simulink model "sscv_braking_ABS_w_vehicle"  (R2024a)
settings: Solver=ode23t  StartTime=0.0  StopTime=1  RelTol=1e-3  AbsTol=1e-3
PreLoadFcn:
  | sscv_braking_ABS_w_vehicle_input
values from neighbouring files (symbols this model uses):
  wheel_rad = 0.3    [sscv_braking_ABS_w_vehicle_input.m]
  wheel_vth = 0.01    [sscv_braking_ABS_w_vehicle_input.m]
undefined symbols (not defined in the file or in its folder): Asphalt, fcdb, HCU, MFormulaCoeff, tpc, vb
libraries: fl_lib x165, SimscapeFluids_lib x24, nesl_utility x21, sdl_lib x9, simulink x3, simulink_extras x1
(part 1 of 6)
CloseFcn:
  | clear brkTs fcdb HCU MFormulaCoeff mu period
  | clear simlog_sscv_braking_ABS_w_vehicle
  | clear Slip tpc tout vb wheel_rad wheel_vth
  | 
  | try,close(h_sscv_braking_ABS_w_vehicle),end
  | clear h_sscv_braking_ABS_w_vehicle
Description:
  | Anti-Lock Braking System (ABS)
settings Model: Creator=The MathWorks, Inc.  LastModifiedBy=The MathWorks, Inc.
settings SolverCC: AutoScaleAbsTol=off  MaxConsecutiveMinStep=10  ZeroCrossAlgorithm=Adaptive  AlgebraicLoopSolver=TrustRegion
settings DataIOCC: SignalLogging=off  ReturnWorkspaceOutputs=off
settings OptimizationCC: ReuseModelBlockBuffer=off
settings DebuggingCC: MaskedZcDiagnostic=none  IgnoredZcDiagnostic=none  UnconnectedInputMsg=warning  UnconnectedOutputMsg=warning  UnconnectedLineMsg=warning
settings ModelReferenceCC: EnableRefExpFcnMdlSchedulingChecks=on
settings RTWCC: GPUComputeCapability=3.5  DLArmComputeVersion=19.05
settings SimscapeCC: SimscapeLogType=all  SimscapeLogName=simlog_sscv_braking_ABS_w_vehicle  SimscapeLogLimitData=off

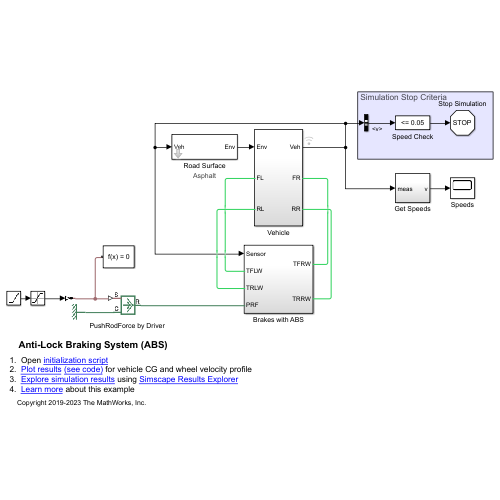
[thumbnail: Simulink's stored preview of the top-level diagram]
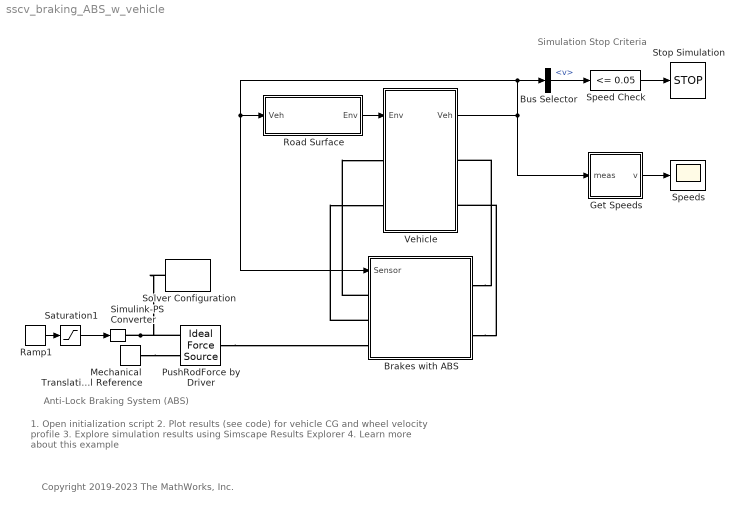
== system sscv_braking_ABS_w_vehicle ==
  note: Anti-Lock Braking System (ABS)
  note: 1. Open initialization script
      | 2. Plot results (see code) for vehicle CG and wheel velocity profile
      | 3. Explore simulation results using Simscape Results Explorer
      | 4. Learn more about this example
  note: Simulation Stop Criteria
  note: Copyright 2019-2023 The MathWorks, Inc.
  Brakes with ABS : Subsystem
  Bus Selector : BusSelector  OutputSignals=v
  Get Speeds : Subsystem
  Mechanical Translational Reference : fl_lib/Mechanical/Translational Elements/Mechanical Translational Reference
  PushRodForce by Driver : fl_lib/Mechanical/Mechanical Sources/Ideal Force Source
  Ramp1 : simulink/Sources/Ramp  slope=tpc.pushRodF(3)*10  start=0.1  InitialOutput=0
  Road Surface : Subsystem  mask{road_condition=Asphalt}
      mask prompts: road_condition "Road Condition"
      settings: AttributesFormatString=%<road_condition>
      mask TypeOptions road_condition: Road/road_condition
  Saturation1 : Saturate  UpperLimit=tpc.pushRodF(3)  LowerLimit=0
  Simulink-PS Converter : nesl_utility/Simulink-PS Converter  PhysicalDomain=network_engine_domain  SubClassName=ps_input  LeftPortType=input  RightPortType=output  PseudoPeriodic=off  Frequencies=[]  NoiseDistribution=none  NoiseParameters=[]  Unit=1  AffineConversion=off  FilteringAndDerivatives=filter  SimscapeFilterOrder=1  InputFilterTimeConstant=0.001  UdotUserProvided=0
  Solver Configuration : nesl_utility/Solver Configuration  Tag=ModelFeatures  PhysicalDomain=network_engine_domain  SubClassName=solver  LeftPortType=input  RightPortType=generic  Tones=[]  Harmonics=[]  SimulateNoise=off  Profile=off  UseLocalSampling=off  EnableSwitchedLinearOptims=on  FrequencyDomain=off  UseCCode=off  RelTol=0.001  AbsTol=1e-06  MinStep=1e-09  ToWorkspace=off  RevertToSquareIcSolve=off  NumHomotopyIterations=100  PhasorMode=off  PhasorModeNumHarmonics=1  ConsistencySolver=NEWTON_FTOL  IndexReductionMethod=DerivativeReplacement  DoDC=off  ResidualTolerance=1e-09  ConsistencyTolSource=GLOBAL  ConsistencyAbsTol=0.001  ConsistencyRelTol=0.001  ConsistencyTolFactor=0.001  UseLocalSolver=off  LocalSolverChoice=NE_BACKWARD_EULER_ADVANCER  ResolveIndetEquations=on  FunctionEvalNumThread=1  LocalSolverSampleTime=0.001  DoFixedCost=off  MaxNonlinIter=3  MaxModeIter=2  ComputeImpulses=off  ImpulseIterations=1  LinearAlgebra=auto  LinearAlgebraNumThread=0  EquationFormulation=NE_TIME_EF  DelaysMemoryBudget=1024  AutomaticFiltering=on  FilteringTimeConstant=0.001  PartitionStorageMethod=AS_NEEDED  PartitionMemoryBudget=1024  PartitionMethod=FAST  MultibodyUseLocalSolver=off  MultibodyLocalSolverChoice=ODE1  MultibodyLocalSolverSampleTime=0.001
  Speed Check : simulink/Logic and Bit Operations/Compare To Constant  relop=<=  const=0.05  OutDataTypeStr=boolean
  Speeds : Scope
  Stop Simulation : Stop
  Vehicle : Subsystem
  wires:
  Speed Check/1 -> Stop Simulation/1
  Vehicle/1(Veh) -> Brakes with ABS/1(Sensor), Road Surface/1(Veh), Bus Selector/1, Get Speeds/1(meas)
  Road Surface/1(Env) -> Vehicle/1(Env)
  Bus Selector/1 -> Speed Check/1  "<v>"
  Get Speeds/1(v) -> Speeds/1
  Ramp1/1 -> Saturation1/1
  Saturation1/1 -> Simulink-PS Converter/1
  connections:
  Brakes with ABS/LConn1 -- Vehicle/LConn1
  Brakes with ABS/RConn1 -- Vehicle/RConn1
  Brakes with ABS/LConn2 -- Vehicle/LConn2
  Brakes with ABS/RConn2 -- Vehicle/RConn2
  Simulink-PS Converter/RConn1 -- PushRodForce by Driver/RConn1 -- Solver Configuration/RConn1
  PushRodForce by Driver/LConn1 -- Brakes with ABS/LConn3
  Mechanical Translational Reference/LConn1 -- PushRodForce by Driver/RConn2

== system sscv_braking_ABS_w_vehicle/Brakes with ABS ==
  note: Fixed Caliper Disc Brakes
  Sensor : Inport
  ABS : Subsystem
  FCDB : Subsystem  Tag=ModelFeatures
  Vacuum Boosted Tandem Primary Cylinder : Subsystem
  TFLW : PMIOPort  Side=Left
  TFRW : PMIOPort  Port=2  Side=Right
  TRLW : PMIOPort  Port=3  Side=Left
  TRRW : PMIOPort  Port=4  Side=Right
  PRF : PMIOPort  Port=5  Side=Left
  wires:
  Sensor/1 -> ABS/1(Sensor)
  connections:
  ABS/LConn3 -- Vacuum Boosted Tandem Primary Cylinder/LConn1
  FCDB/LConn3 -- ABS/LConn1
  FCDB/RConn2 -- TRRW/RConn1
  ABS/LConn2 -- FCDB/LConn4
  ABS/RConn2 -- FCDB/RConn4
  FCDB/RConn3 -- ABS/RConn1
  ABS/RConn3 -- Vacuum Boosted Tandem Primary Cylinder/RConn1
  FCDB/RConn1 -- TFRW/RConn1
  FCDB/LConn1 -- TFLW/RConn1
  FCDB/LConn2 -- TRLW/RConn1
  PRF/RConn1 -- Vacuum Boosted Tandem Primary Cylinder/LConn2

== system sscv_braking_ABS_w_vehicle/Get Speeds ==
  meas : Inport
  Bus Selector2 : BusSelector  OutputSignals=v,FL.v,FR.v,RL.v,RR.v
  Demux : Demux  Outputs=5
  Mux : Mux  Inputs=5
  Mux1 : Mux  Inputs=5
  v : Outport  VectorParamsAs1DForOutWhenUnconnected=off
  wires:
  Bus Selector2/4 -> Mux/4  "<v>"
  Bus Selector2/3 -> Mux/3  "<v>"
  Bus Selector2/2 -> Mux/2  "<v>"
  Bus Selector2/5 -> Mux/5  "<v>"
  meas/1 -> Bus Selector2/1
  Bus Selector2/1 -> Mux/1  "<v>"
  Mux/1 -> Demux/1
  Mux1/1 -> v/1
  Demux/1 -> Mux1/1  "Vehicle CG  velocity"
  Demux/2 -> Mux1/2  "Front left tire velocity"
  Demux/3 -> Mux1/3  "Front right tire velocity"
  Demux/4 -> Mux1/4  "Rear left tire velocity"
  Demux/5 -> Mux1/5  "Rear right tire velocity"

== system sscv_braking_ABS_w_vehicle/Road Surface ==
  In Bus Element : Inport  PortName=Veh  Element=x
  Bus Creator : BusCreator  Inputs=3
  Bus Creator1 : BusCreator  Inputs=4
  Constant : Constant  Value=0
  Constant1 : Constant  Value=0
  Road : Subsystem  mask(Testing Surface){road_condition=Asphalt, surface_LF=0, surface_RF=0, surface_LR=0, surface_RR=0, surface_xpos=0}
      mask prompts: road_condition "Road Condition"; surface_LF "Surface LF"; surface_RF "Surface RF"; surface_LR "Surface LR"; surface_RR "Surface RR"; surface_xpos "Surface Position"
      mask help: Select surface for test. Specifies locations of high and low friction surface as a function of longitudinal distance for each tire.
      mask init:
      | if (road_condition==1)
      |     % Road: low coeff to high coeff
      |     surface_LF   = [3 1 1 3 3];
      |     surface_RF   = [3 1 1 3 3];
      |     surface_LR   = [3 1 1 3 3];
      |     surface_RR   = [3 1 1 3 3];
      |     surface_xpos = [-1 0 24.9 25 26]+6;
      | elseif(road_condition==2)
      |     % Road: Split (low left side)
      |     surface_LF   = [1 1 1 1 1];
      |     surface_RF   = [4 4 4 4 4];
      |     surface_LR   = [1 1 1 1 1];
      |     surface_RR   = [4 4 4 4 4];
      |     surface_xpos = [-1 0 4.9 5 6];
      | elseif(road_condition==3)
      |     % Road: Asphalt
      |     surface_LF   = [4 4 4 4 4];
      |     surface_RF   = [4 4 4 4 4];
      |     surface_LR   = [4 4 4 4 4];
      |     surface_RR   = [4 4 4 4 4];
      |     surface_xpos = [-1 0 4.9 5 6];
      | elseif(road_condition==4)
      |     % Road: Wet Asphalt
      |     surface_LF   = [3 3 3 3 3];
      |     surface_RF   = [3 3 3 3 3];
      |     surface_LR   = [3 3 3 3 3];
      |     surface_RR   = [3 3 3 3 3];
      |     surface_xpos = [-1 0 4.9 5 6];
      | elseif(road_condition==5)
      |     % Road: Ice
      |     surface_LF   = [1 1 1 1 1];
      |     surface_RF   = [1 1 1 1 1];
      |     surface_LR   = [1 1 1 1 1];
      |     surface_RR   = [1 1 1 1 1];
      |     surface_xpos = [-1 0 4.9 5 6];
      | end
      settings: AttributesFormatString=%<road_condition>
      mask TypeOptions road_condition: Transition: Low to high mu | Split: Low mu on left | Asphalt | Wet Asphalt | Ice
  Env : Outport  VectorParamsAs1DForOutWhenUnconnected=off
  wires:
  Constant1/1 -> Bus Creator/2  "Slope"
  Constant/1 -> Bus Creator/1  "Wind"
  Bus Creator/1 -> Env/1  "Env"
  Road/1(FL) -> Bus Creator1/1  "FL"
  Road/2(FR) -> Bus Creator1/2  "FR"
  Road/3(RL) -> Bus Creator1/3  "RL"
  Road/4(RR) -> Bus Creator1/4  "RR"
  Bus Creator1/1 -> Bus Creator/3  "mu"
  In Bus Element/1 -> Road/1(wX)

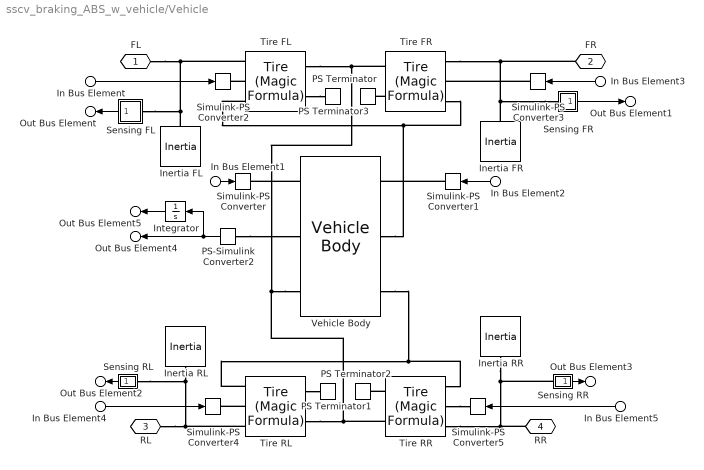
== system sscv_braking_ABS_w_vehicle/Vehicle ==
  In Bus Element1 : Inport  PortName=Env  Element=Wind
  In Bus Element2 : Inport  PortName=Env  Element=Slope
  In Bus Element : Inport  PortName=Env  Element=mu.FL
  In Bus Element3 : Inport  PortName=Env  Element=mu.FR
  In Bus Element4 : Inport  PortName=Env  Element=mu.RL
  In Bus Element5 : Inport  PortName=Env  Element=mu.RR
  Inertia FL : fl_lib/Mechanical/Rotational Elements/Inertia  inertia=0.36728 kg*m^2  num_ports=foundation.enum.numPorts2.one  w_specify=on  w_priority=Low  w=100e3/3600/0.3 rad/s  w_nominal_specify=off  w_nominal_value=1  w_nominal_unit=rad/s  t_specify=off  t_priority=High  t=0 N*m  t_nominal_specify=off  t_nominal_value=1  t_nominal_unit=N*m
  Inertia FR : fl_lib/Mechanical/Rotational Elements/Inertia  inertia=0.36728 kg*m^2  num_ports=foundation.enum.numPorts2.one  w_specify=on  w_priority=Low  w=100e3/3600/0.3 rad/s  w_nominal_specify=off  w_nominal_value=1  w_nominal_unit=rad/s  t_specify=off  t_priority=High  t=0 N*m  t_nominal_specify=off  t_nominal_value=1  t_nominal_unit=N*m
  Inertia RL : fl_lib/Mechanical/Rotational Elements/Inertia  inertia=0.36728 kg*m^2  num_ports=foundation.enum.numPorts2.one  w_specify=on  w_priority=Low  w=100e3/3600/0.3 rad/s  w_nominal_specify=off  w_nominal_value=1  w_nominal_unit=rad/s  t_specify=off  t_priority=High  t=0 N*m  t_nominal_specify=off  t_nominal_value=1  t_nominal_unit=N*m
  Inertia RR : fl_lib/Mechanical/Rotational Elements/Inertia  inertia=0.36728 kg*m^2  num_ports=foundation.enum.numPorts2.one  w_specify=on  w_priority=Low  w=100e3/3600/0.3 rad/s  w_nominal_specify=off  w_nominal_value=1  w_nominal_unit=rad/s  t_specify=off  t_priority=High  t=0 N*m  t_nominal_specify=off  t_nominal_value=1  t_nominal_unit=N*m
  Integrator : Integrator  InitialCondition=[0 0 0 0]
  PS Terminator{,1..3} (4 alike) : fl_lib/Physical Signals/Sinks/PS Terminator
  PS-Simulink Converter2 : nesl_utility/PS-Simulink Converter  PhysicalDomain=network_engine_domain  SubClassName=ps_output  LeftPortType=input  RightPortType=output  PseudoPeriodic=off  Frequencies=[]  VectorFormat=1-D array  Unit=m/s  AffineConversion=off
  Sensing FL : Subsystem
      mask Display: disp('w')
  Sensing FR : Subsystem
      mask Display: disp('w')
  Sensing RL : Subsystem
      mask Display: disp('w')
  Sensing RR : Subsystem
      mask Display: disp('w')
  Simulink-PS Converter{,1..5} (6 alike) : nesl_utility/Simulink-PS Converter  PhysicalDomain=network_engine_domain  SubClassName=ps_input  LeftPortType=input  RightPortType=output  PseudoPeriodic=off  Frequencies=[]  NoiseDistribution=none  NoiseParameters=[]  Unit=1  AffineConversion=off  FilteringAndDerivatives=provide  SimscapeFilterOrder=1  InputFilterTimeConstant=0.001  UdotUserProvided=0
  Tire FL : sdl_lib/Tires & Vehicles/Tire (Magic Formula)  parameterization=4  F_z1=3000 N  F_x1=3500 N  kappa1=10  B_m=10  C_m=1.9  D_m=1  E_m=0.97  fz0=4000 N  p_Cx=1.685  p_Dx=[1.21, -.037]  p_Ex=[.344, .095, -.02, 0]  p_Kx=[21.51, -.163, .245]  p_Hx=[-.002, .002]  p_Vx=[0, 0]  rolling_radius_model=sdl.enum.RollingRadiusParameterization.Constant  r_e=wheel_rad m  r_0=0.3 m  breff=8.39  dreff=0.26  freff=0.074  q_re0=0.99  q_v1=0.008  longvl=17 m/s  cz=5e5 N/m  model_resistance=0  resistance_model=1  coeff=0.015  p_tire=250e3 Pa  alpha=-0.003  beta=0.97  coeff_a=84e-4  coeff_b=6.2e-4 s/m  coeff_c=1.6e-4 s^2/m^2  p_tire0=240e3 Pa  fz0_resistance=4000 N  vH0=16 m/s  q_Sy=[.0082, 0, .0014, .001, 0, 0, 1.08, -.5]  v_thr=0.001 m/s  enable_scaling_coefficients=false  lfzO=1  lcx=1  lmux=1  lex=1  lkx=1  lhx=1  lvx=1  lmy=1  model_compliance=0  stiffness=1e6 N/m  damping=1000 N/(m/s)  model_inertia=0  inertia=1 kg*m^2  initial_velocity=0 rad/s  vxlow=wheel_vth m/s  v_tr_thr=0.1*(wheel_vth) m/s  kpumin=-1e5  kpumax=1e5
      settings: InternalSimscapePortConfiguration="{\"Bottom\":[],\"Left\":[{\"id\":\"N\",\"label\":\"N\",\"type\":\"input\"},{\"id\":\"M\",\"label\":\"M\",\"type\":\"input\"},{\"id\":\"A\",\"label\":\"A\",\"type\":\"foundation.mechanical.rotational.rotational\"}],\"Right\":[{\"id\":\"S\",\"label\":\"S\",\"type\":\"output\"},{\"id\":\"H\",\"label\":\"H\",\"type\":\"foundation.mechanical.translational.translational\"}],\"Top\":[]}"
  Tire FR : sdl_lib/Tires & Vehicles/Tire (Magic Formula)  parameterization=4  F_z1=3000 N  F_x1=3500 N  kappa1=10  B_m=10  C_m=1.9  D_m=1  E_m=0.97  fz0=4000 N  p_Cx=1.685  p_Dx=[1.21, -.037]  p_Ex=[.344, .095, -.02, 0]  p_Kx=[21.51, -.163, .245]  p_Hx=[-.002, .002]  p_Vx=[0, 0]  rolling_radius_model=sdl.enum.RollingRadiusParameterization.Constant  r_e=wheel_rad m  r_0=0.3 m  breff=8.39  dreff=0.26  freff=0.074  q_re0=0.99  q_v1=0.008  longvl=17 m/s  cz=5e5 N/m  model_resistance=0  resistance_model=1  coeff=0.015  p_tire=250e3 Pa  alpha=-0.003  beta=0.97  coeff_a=84e-4  coeff_b=6.2e-4 s/m  coeff_c=1.6e-4 s^2/m^2  p_tire0=240e3 Pa  fz0_resistance=4000 N  vH0=16 m/s  q_Sy=[.0082, 0, .0014, .001, 0, 0, 1.08, -.5]  v_thr=0.001 m/s  enable_scaling_coefficients=false  lfzO=1  lcx=1  lmux=1  lex=1  lkx=1  lhx=1  lvx=1  lmy=1  model_compliance=0  stiffness=1e6 N/m  damping=1000 N/(m/s)  model_inertia=0  inertia=1 kg*m^2  initial_velocity=0 rad/s  vxlow=wheel_vth m/s  v_tr_thr=0.1*(wheel_vth) m/s  kpumin=-1e5  kpumax=1e5
      settings: InternalSimscapePortConfiguration="{\"Bottom\":[],\"Left\":[{\"id\":\"N\",\"label\":\"N\",\"type\":\"input\"},{\"id\":\"M\",\"label\":\"M\",\"type\":\"input\"},{\"id\":\"A\",\"label\":\"A\",\"type\":\"foundation.mechanical.rotational.rotational\"}],\"Right\":[{\"id\":\"S\",\"label\":\"S\",\"type\":\"output\"},{\"id\":\"H\",\"label\":\"H\",\"type\":\"foundation.mechanical.translational.translational\"}],\"Top\":[]}"
  Tire RL : sdl_lib/Tires & Vehicles/Tire (Magic Formula)  parameterization=4  F_z1=3000 N  F_x1=3500 N  kappa1=10  B_m=10  C_m=1.9  D_m=1  E_m=0.97  fz0=4000 N  p_Cx=1.685  p_Dx=[1.21, -.037]  p_Ex=[.344, .095, -.02, 0]  p_Kx=[21.51, -.163, .245]  p_Hx=[-.002, .002]  p_Vx=[0, 0]  rolling_radius_model=sdl.enum.RollingRadiusParameterization.Constant  r_e=wheel_rad m  r_0=0.3 m  breff=8.39  dreff=0.26  freff=0.074  q_re0=0.99  q_v1=0.008  longvl=17 m/s  cz=5e5 N/m  model_resistance=0  resistance_model=1  coeff=0.015  p_tire=250e3 Pa  alpha=-0.003  beta=0.97  coeff_a=84e-4  coeff_b=6.2e-4 s/m  coeff_c=1.6e-4 s^2/m^2  p_tire0=240e3 Pa  fz0_resistance=4000 N  vH0=16 m/s  q_Sy=[.0082, 0, .0014, .001, 0, 0, 1.08, -.5]  v_thr=0.001 m/s  enable_scaling_coefficients=false  lfzO=1  lcx=1  lmux=1  lex=1  lkx=1  lhx=1  lvx=1  lmy=1  model_compliance=0  stiffness=1e6 N/m  damping=1000 N/(m/s)  model_inertia=0  inertia=1 kg*m^2  initial_velocity=0 rad/s  vxlow=wheel_vth m/s  v_tr_thr=0.1*(wheel_vth) m/s  kpumin=-1e5  kpumax=1e5
      settings: InternalSimscapePortConfiguration="{\"Bottom\":[],\"Left\":[{\"id\":\"N\",\"label\":\"N\",\"type\":\"input\"},{\"id\":\"M\",\"label\":\"M\",\"type\":\"input\"},{\"id\":\"A\",\"label\":\"A\",\"type\":\"foundation.mechanical.rotational.rotational\"}],\"Right\":[{\"id\":\"S\",\"label\":\"S\",\"type\":\"output\"},{\"id\":\"H\",\"label\":\"H\",\"type\":\"foundation.mechanical.translational.translational\"}],\"Top\":[]}"
  Tire RR : sdl_lib/Tires & Vehicles/Tire (Magic Formula)  parameterization=4  F_z1=3000 N  F_x1=3500 N  kappa1=10  B_m=10  C_m=1.9  D_m=1  E_m=0.97  fz0=4000 N  p_Cx=1.685  p_Dx=[1.21, -.037]  p_Ex=[.344, .095, -.02, 0]  p_Kx=[21.51, -.163, .245]  p_Hx=[-.002, .002]  p_Vx=[0, 0]  rolling_radius_model=sdl.enum.RollingRadiusParameterization.Constant  r_e=wheel_rad m  r_0=0.3 m  breff=8.39  dreff=0.26  freff=0.074  q_re0=0.99  q_v1=0.008  longvl=17 m/s  cz=5e5 N/m  model_resistance=0  resistance_model=1  coeff=0.015  p_tire=250e3 Pa  alpha=-0.003  beta=0.97  coeff_a=84e-4  coeff_b=6.2e-4 s/m  coeff_c=1.6e-4 s^2/m^2  p_tire0=240e3 Pa  fz0_resistance=4000 N  vH0=16 m/s  q_Sy=[.0082, 0, .0014, .001, 0, 0, 1.08, -.5]  v_thr=0.001 m/s  enable_scaling_coefficients=false  lfzO=1  lcx=1  lmux=1  lex=1  lkx=1  lhx=1  lvx=1  lmy=1  model_compliance=0  stiffness=1e6 N/m  damping=1000 N/(m/s)  model_inertia=0  inertia=1 kg*m^2  initial_velocity=0 rad/s  vxlow=wheel_vth m/s  v_tr_thr=0.1*(wheel_vth) m/s  kpumin=-1e5  kpumax=1e5
      settings: InternalSimscapePortConfiguration="{\"Bottom\":[],\"Left\":[{\"id\":\"N\",\"label\":\"N\",\"type\":\"input\"},{\"id\":\"M\",\"label\":\"M\",\"type\":\"input\"},{\"id\":\"A\",\"label\":\"A\",\"type\":\"foundation.mechanical.rotational.rotational\"}],\"Right\":[{\"id\":\"S\",\"label\":\"S\",\"type\":\"output\"},{\"id\":\"H\",\"label\":\"H\",\"type\":\"foundation.mechanical.translational.translational\"}],\"Top\":[]}"
  Vehicle Body : sdl_lib/Tires & Vehicles/Vehicle Body  mass=1500 kg  n_w=2  x_f=1.4 m  x_r=1.6 m  y_c=0.5 m  mass_var=simscape.enum.onoff.off  g=9.81 m/s^2  liftoff_warning=simscape.enum.onoff.off  area=1 m^2  Cd=0.25  rho=1.18 kg/m^3  model_pitch=simscape.enum.onoff.off  inertia=4000 kg*m^2  suspension_model=sdl.enum.linearTLU.linear  k_f=1e4 N/m  b_f=1e4 N/(m/s)  k_r=1e4 N/m  b_r=1e4 N/(m/s)  k_f_TLU=[-2000, -1000, 0, 1000, 2000] N  x_f_TLU=[-.4, -.2, 0, .2, .4] m  b_f_TLU=[-200, -100, 0, 100, 200] N  v_f_TLU=[-4, -2, 0, 2, 4] m/s  k_r_TLU=[-2000, -1000, 0, 1000, 2000] N  x_r_TLU=[-.4, -.2, 0, .2, .4] m  b_r_TLU=[-200, -100, 0, 100, 200] N  v_r_TLU=[-4, -2, 0, 2, 4] m/s  interp_method=simscape.enum.interpolation.linear  extrap_method=simscape.enum.extrapolation.linear  model_hardstop=simscape.enum.onoff.off  upper_bound_f=.25 m  lower_bound_f=-.25 m  stop_k_f=1e6 N/m  stop_b_f=150 N/(m/s)  upper_bound_r=.25 m  lower_bound_r=-.25 m  stop_k_r=1e6 N/m  stop_b_r=150 N/(m/s)  initial_pitch=0 rad  initial_pitch_rate=0 rad/s  v_specify=on  v_priority=High  v=100 km/hr  v_nominal_specify=off  v_nominal_value=1  v_nominal_unit=m/s
  FL : PMIOPort  Side=Left
  FR : PMIOPort  Port=2  Side=Right
  RL : PMIOPort  Port=3  Side=Left
  RR : PMIOPort  Port=4  Side=Right
  Out Bus Element4 : Outport  VectorParamsAs1DForOutWhenUnconnected=off  PortName=Veh  Element=v
  Out Bus Element : Outport  VectorParamsAs1DForOutWhenUnconnected=off  PortName=Veh  Element=FL.v
  Out Bus Element1 : Outport  VectorParamsAs1DForOutWhenUnconnected=off  PortName=Veh  Element=FR.v
  Out Bus Element5 : Outport  VectorParamsAs1DForOutWhenUnconnected=off  PortName=Veh  Element=x
  Out Bus Element2 : Outport  VectorParamsAs1DForOutWhenUnconnected=off  PortName=Veh  Element=RL.v
  Out Bus Element3 : Outport  VectorParamsAs1DForOutWhenUnconnected=off  PortName=Veh  Element=RR.v
  wires:
  Sensing RR/1(w) -> Out Bus Element3/1
  Sensing RL/1(w) -> Out Bus Element2/1
  Sensing FL/1(w) -> Out Bus Element/1
  Sensing FR/1(w) -> Out Bus Element1/1
  In Bus Element2/1 -> Simulink-PS Converter1/1
  In Bus Element1/1 -> Simulink-PS Converter/1
  In Bus Element3/1 -> Simulink-PS Converter3/1
  In Bus Element/1 -> Simulink-PS Converter2/1
  In Bus Element4/1 -> Simulink-PS Converter4/1
  In Bus Element5/1 -> Simulink-PS Converter5/1
  PS-Simulink Converter2/1 -> Integrator/1, Out Bus Element4/1
  Integrator/1 -> Out Bus Element5/1
  connections:
  Sensing FR/LConn1 -- Inertia FR/LConn1 -- Tire FR/LConn3 -- FR/RConn1
  Simulink-PS Converter1/RConn1 -- Vehicle Body/RConn3
  RR/RConn1 -- Sensing RR/LConn1 -- Inertia RR/LConn1 -- Tire RR/LConn3
  PS-Simulink Converter2/LConn1 -- Vehicle Body/LConn2
  Sensing FL/LConn1 -- Tire FL/LConn3 -- FL/RConn1 -- Inertia FL/LConn1
  Vehicle Body/LConn1 -- Tire RR/RConn2 -- Tire RL/RConn2 -- Tire FL/RConn2 -- Tire FR/RConn2
  Tire RR/RConn1 -- PS Terminator1/LConn1
  Tire RL/RConn1 -- PS Terminator2/LConn1
  Tire FR/RConn1 -- PS Terminator/LConn1
  Tire FL/RConn1 -- PS Terminator3/LConn1
  Vehicle Body/LConn3 -- Simulink-PS Converter/RConn1
  Vehicle Body/RConn1 -- Tire RL/LConn1 -- Tire RR/LConn1
  Vehicle Body/RConn2 -- Tire FL/LConn1 -- Tire FR/LConn1
  RL/RConn1 -- Tire RL/LConn3 -- Sensing RL/LConn1 -- Inertia RL/LConn1
  Tire FL/LConn2 -- Simulink-PS Converter2/RConn1
  Tire RL/LConn2 -- Simulink-PS Converter4/RConn1
  Tire RR/LConn2 -- Simulink-PS Converter5/RConn1
  Simulink-PS Converter3/RConn1 -- Tire FR/LConn2

== system sscv_braking_ABS_w_vehicle/Brakes with ABS/ABS ==
  note: Hydraulic Control Unit
  Sensor : Inport
  ECU : Subsystem  VariantControl=Control
  HCU : Subsystem
  FR : PMIOPort  Side=Right
  FL : PMIOPort  Port=2  Side=Left
  RL : PMIOPort  Port=3  Side=Left
  RR : PMIOPort  Port=4  Side=Right
  Brk1 : PMIOPort  Port=5  Side=Left
  Brk2 : PMIOPort  Port=6  Side=Right
  wires:
  ECU/1(Valves) -> HCU/1(Valve)
  Sensor/1 -> ECU/1(Sensor)
  connections:
  Brk1/RConn1 -- HCU/LConn1
  Brk2/RConn1 -- HCU/LConn2
  HCU/RConn1 -- FR/RConn1
  HCU/RConn2 -- FL/RConn1
  HCU/RConn3 -- RR/RConn1
  HCU/RConn4 -- RL/RConn1

== system sscv_braking_ABS_w_vehicle/Brakes with ABS/FCDB ==
  FLW : Subsystem
      mask Display:
      | image('sscv_braking_caliper_disk_brake.png');
      | port_label('LConn',1,'Brk1')
      | port_label('RConn',1,'TFLW')
  FRW : Subsystem
      mask Display:
      | image('sscv_braking_caliper_disk_brake.png');
      | port_label('LConn',1,'Brk1')
      | port_label('RConn',1,'TFRW')
  RLW : Subsystem
      mask Display:
      | image('sscv_braking_caliper_disk_brake.png');
      | port_label('LConn',1,'Brk2')
      | port_label('RConn',1,'TRLW')
  RRW : Subsystem
      mask Display:
      | image('sscv_braking_caliper_disk_brake.png');
      | port_label('LConn',1,'Brk2')
      | port_label('RConn',1,'TRRW')
  TFLW : PMIOPort  Side=Left
  TFRW : PMIOPort  Port=2  Side=Right
  TRLW : PMIOPort  Port=3  Side=Left
  FL : PMIOPort  Port=4  Side=Left
  TRRW : PMIOPort  Port=5  Side=Right
  FR : PMIOPort  Port=6  Side=Right
  RR : PMIOPort  Port=7  Side=Right
  RL : PMIOPort  Port=8  Side=Left
  connections:
  FRW/RConn1 -- TFRW/RConn1
  FLW/RConn1 -- TFLW/RConn1
  RRW/RConn1 -- TRRW/RConn1
  RLW/RConn1 -- TRLW/RConn1
  FR/RConn1 -- FRW/LConn1
  FL/RConn1 -- FLW/LConn1
  RR/RConn1 -- RRW/LConn1
  RL/RConn1 -- RLW/LConn1

== system sscv_braking_ABS_w_vehicle/Brakes with ABS/Vacuum Boosted Tandem Primary Cylinder ==
  note: Vacuum Booster
  note: Tandem Primary Cylinder
  TPC : Subsystem
      mask Display:
      | image('sscv_braking_tandem_primary_cylinder.png');
      | port_label('LConn',1,'Brk1')
      | port_label('LConn',2,'Brk2')
      | port_label('RConn',1,'PRF')
  VB : Subsystem  Tag=ModelFeatures
      mask Display:
      | image('sscv_braking_vacuum_booster.png');
      | port_label('LConn',1,'PRF')
      | port_label('RConn',1,'Ftransfer')
  Brk1 : PMIOPort  Side=Left
  PRF : PMIOPort  Port=2  Side=Left
  Brk2 : PMIOPort  Port=3  Side=Right
  connections:
  TPC/RConn1 -- VB/RConn1
  PRF/RConn1 -- VB/LConn1
  TPC/LConn2 -- Brk2/RConn1
  TPC/LConn1 -- Brk1/RConn1

== system sscv_braking_ABS_w_vehicle/Road Surface/Road ==
  note: Wheel position is converted by the
      | lookup table to an integer
      | that indicates the road condition.
  note: The road condition integer is used to select
      | a set of Magic Formula coefficients
      | that correspond to tire behavior on that surface.
  wX : Inport
  Demux : Demux
  Mux : Mux
  Position to Surface LF : Lookup_n-D  NumberOfTableDimensions=1  LookupTableObject=''  BreakpointsForDimension1=surface_xpos  BeginIndexSearchUsingPreviousIndexResult=on  Table=surface_LF  InterpMethod=Flat  InternalRulePriority=Speed  RndMeth=Simplest
  Position to Surface LR : Lookup_n-D  NumberOfTableDimensions=1  LookupTableObject=''  BreakpointsForDimension1=surface_xpos  BeginIndexSearchUsingPreviousIndexResult=on  Table=surface_LR  InterpMethod=Flat  InternalRulePriority=Speed  RndMeth=Simplest
  Position to Surface RF1 : Lookup_n-D  NumberOfTableDimensions=1  LookupTableObject=''  BreakpointsForDimension1=surface_xpos  BeginIndexSearchUsingPreviousIndexResult=on  Table=surface_RF  InterpMethod=Flat  InternalRulePriority=Speed  RndMeth=Simplest
  Position to Surface RR : Lookup_n-D  NumberOfTableDimensions=1  LookupTableObject=''  BreakpointsForDimension1=surface_xpos  BeginIndexSearchUsingPreviousIndexResult=on  Table=surface_RR  InterpMethod=Flat  InternalRulePriority=Speed  RndMeth=Simplest
  Scope : Scope  NumInputPorts=2
  Select MF Coefficients : Subsystem
  FL : Outport  VectorParamsAs1DForOutWhenUnconnected=off
  FR : Outport  Port=2  VectorParamsAs1DForOutWhenUnconnected=off
  RL : Outport  Port=3  VectorParamsAs1DForOutWhenUnconnected=off
  RR : Outport  Port=4  VectorParamsAs1DForOutWhenUnconnected=off
  wires:
  Select MF Coefficients/3(LR) -> RL/1
  Select MF Coefficients/4(RR) -> RR/1
  Select MF Coefficients/1(LF) -> FL/1
  Select MF Coefficients/2(RF) -> FR/1
  wX/1 -> Scope/1, Demux/1  "WhlX"
  Mux/1 -> Scope/2, Select MF Coefficients/1(Surface)
  Demux/1 -> Position to Surface LF/1
  Position to Surface LF/1 -> Mux/1
  Position to Surface RR/1 -> Mux/4
  Demux/4 -> Position to Surface RR/1
  Demux/2 -> Position to Surface RF1/1
  Position to Surface RF1/1 -> Mux/2
  Position to Surface LR/1 -> Mux/3
  Demux/3 -> Position to Surface LR/1

== system sscv_braking_ABS_w_vehicle/Vehicle/Sensing FL ==
  Gain : Gain  Gain=wheel_rad
  Mechanical Rotational Reference : fl_lib/Mechanical/Rotational Elements/Mechanical Rotational Reference
  Motion Sensor : fl_lib/Mechanical/Mechanical Sensors/Ideal Rotational Motion Sensor  reference=foundation.enum.MeasurementReference.difference  acceleration_port=false  velocity_port=true  position_port=true  wrap_angle=simscape.enum.onoff.off  offset=0 rad
  PS Terminator4 : fl_lib/Physical Signals/Sinks/PS Terminator
  PS-Simulink Converter : nesl_utility/PS-Simulink Converter  PhysicalDomain=network_engine_domain  SubClassName=ps_output  LeftPortType=input  RightPortType=output  PseudoPeriodic=off  Frequencies=[]  VectorFormat=1-D array  Unit=1  AffineConversion=off
  R : PMIOPort  Side=Left
  w : Outport  VectorParamsAs1DForOutWhenUnconnected=off
  wires:
  PS-Simulink Converter/1 -> Gain/1
  Gain/1 -> w/1
  connections:
  Motion Sensor/RConn2 -- PS-Simulink Converter/LConn1
  Motion Sensor/RConn3 -- PS Terminator4/LConn1
  Motion Sensor/RConn1 -- Mechanical Rotational Reference/LConn1
  R/RConn1 -- Motion Sensor/LConn1

== system sscv_braking_ABS_w_vehicle/Vehicle/Sensing FR ==
  Gain : Gain  Gain=wheel_rad
  Mechanical Rotational Reference : fl_lib/Mechanical/Rotational Elements/Mechanical Rotational Reference
  Motion Sensor : fl_lib/Mechanical/Mechanical Sensors/Ideal Rotational Motion Sensor  reference=foundation.enum.MeasurementReference.difference  acceleration_port=false  velocity_port=true  position_port=true  wrap_angle=simscape.enum.onoff.off  offset=0 rad
  PS Terminator4 : fl_lib/Physical Signals/Sinks/PS Terminator
  PS-Simulink Converter : nesl_utility/PS-Simulink Converter  PhysicalDomain=network_engine_domain  SubClassName=ps_output  LeftPortType=input  RightPortType=output  PseudoPeriodic=off  Frequencies=[]  VectorFormat=1-D array  Unit=1  AffineConversion=off
  R : PMIOPort  Side=Left
  w : Outport  VectorParamsAs1DForOutWhenUnconnected=off
  wires:
  Gain/1 -> w/1
  PS-Simulink Converter/1 -> Gain/1
  connections:
  R/RConn1 -- Motion Sensor/LConn1
  Motion Sensor/RConn1 -- Mechanical Rotational Reference/LConn1
  Motion Sensor/RConn3 -- PS Terminator4/LConn1
  Motion Sensor/RConn2 -- PS-Simulink Converter/LConn1

== system sscv_braking_ABS_w_vehicle/Vehicle/Sensing RL ==
  Gain : Gain  Gain=wheel_rad
  Mechanical Rotational Reference : fl_lib/Mechanical/Rotational Elements/Mechanical Rotational Reference
  Motion Sensor : fl_lib/Mechanical/Mechanical Sensors/Ideal Rotational Motion Sensor  reference=foundation.enum.MeasurementReference.difference  acceleration_port=false  velocity_port=true  position_port=true  wrap_angle=simscape.enum.onoff.off  offset=0 rad
  PS Terminator4 : fl_lib/Physical Signals/Sinks/PS Terminator
  PS-Simulink Converter : nesl_utility/PS-Simulink Converter  PhysicalDomain=network_engine_domain  SubClassName=ps_output  LeftPortType=input  RightPortType=output  PseudoPeriodic=off  Frequencies=[]  VectorFormat=1-D array  Unit=1  AffineConversion=off
  R : PMIOPort  Side=Left
  w : Outport  VectorParamsAs1DForOutWhenUnconnected=off
  wires:
  Gain/1 -> w/1
  PS-Simulink Converter/1 -> Gain/1
  connections:
  R/RConn1 -- Motion Sensor/LConn1
  Motion Sensor/RConn1 -- Mechanical Rotational Reference/LConn1
  Motion Sensor/RConn3 -- PS Terminator4/LConn1
  Motion Sensor/RConn2 -- PS-Simulink Converter/LConn1

== system sscv_braking_ABS_w_vehicle/Vehicle/Sensing RR ==
  Gain : Gain  Gain=wheel_rad
  Mechanical Rotational Reference : fl_lib/Mechanical/Rotational Elements/Mechanical Rotational Reference
  Motion Sensor : fl_lib/Mechanical/Mechanical Sensors/Ideal Rotational Motion Sensor  reference=foundation.enum.MeasurementReference.difference  acceleration_port=false  velocity_port=true  position_port=true  wrap_angle=simscape.enum.onoff.off  offset=0 rad
  PS Terminator4 : fl_lib/Physical Signals/Sinks/PS Terminator
  PS-Simulink Converter : nesl_utility/PS-Simulink Converter  PhysicalDomain=network_engine_domain  SubClassName=ps_output  LeftPortType=input  RightPortType=output  PseudoPeriodic=off  Frequencies=[]  VectorFormat=1-D array  Unit=1  AffineConversion=off
  R : PMIOPort  Side=Left
  w : Outport  VectorParamsAs1DForOutWhenUnconnected=off
  wires:
  PS-Simulink Converter/1 -> Gain/1
  Gain/1 -> w/1
  connections:
  Motion Sensor/RConn2 -- PS-Simulink Converter/LConn1
  Motion Sensor/RConn3 -- PS Terminator4/LConn1
  Motion Sensor/RConn1 -- Mechanical Rotational Reference/LConn1
  R/RConn1 -- Motion Sensor/LConn1

== system sscv_braking_ABS_w_vehicle/Brakes with ABS/ABS/ECU ==
  Sensor : Inport
  Bus Creator : BusCreator  Inputs=4
  Bus Selector : BusSelector  OutputSignals=FL
  Bus Selector1 : BusSelector  OutputSignals=FR
  Bus Selector2 : BusSelector  OutputSignals=RL
  Bus Selector3 : BusSelector  OutputSignals=RR
  Calculate Slip : Subsystem
  Valve Control FL : Subsystem
  Valve Control FR : Subsystem
  Valve Control RL : Subsystem
  Valve Control RR : Subsystem
  Vehicle Speed : Subsystem
  Valves : Outport  VectorParamsAs1DForOutWhenUnconnected=off
  wires:
  Sensor/1 -> Vehicle Speed/1(Sensors), Calculate Slip/1(WhlSpd)
  Vehicle Speed/1(vSpdEst) -> Valve Control FR/2(vSpdEst), Valve Control RL/2(vSpdEst), Valve Control RR/2(vSpdEst), Valve Control FL/2(vSpdEst), Calculate Slip/2(VehSpdEst)
  Calculate Slip/1(Slip) -> Bus Selector3/1, Bus Selector2/1, Bus Selector1/1, Bus Selector/1
  Bus Selector/1 -> Valve Control FL/1(Slip)  "<FL>"
  Bus Creator/1 -> Valves/1  "Valves"
  Bus Selector1/1 -> Valve Control FR/1(Slip)  "<FR>"
  Bus Selector2/1 -> Valve Control RL/1(Slip)  "<RL>"
  Bus Selector3/1 -> Valve Control RR/1(Slip)  "<RR>"
  Valve Control FL/1(Valve) -> Bus Creator/1  "FL"
  Valve Control FR/1(Valve) -> Bus Creator/2  "FR"
  Valve Control RL/1(Valve) -> Bus Creator/3  "RL"
  Valve Control RR/1(Valve) -> Bus Creator/4  "RR"

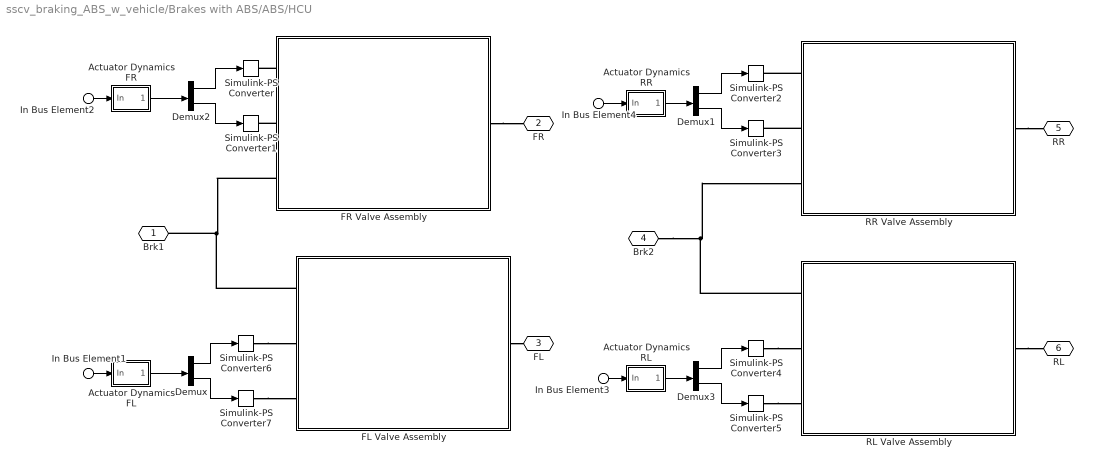
== system sscv_braking_ABS_w_vehicle/Brakes with ABS/ABS/HCU ==
  In Bus Element4 : Inport  PortName=Valve  Element=RR
  In Bus Element2 : Inport  PortName=Valve  Element=FR
  In Bus Element1 : Inport  PortName=Valve  Element=FL
  In Bus Element3 : Inport  PortName=Valve  Element=RL
  Actuator Dynamics FL : Subsystem  mask(First-order lag supporting vector signals){b=HCU.brkTs, x_initial=0}
      mask prompts: b "Filter time constant"; x_initial "Initial output"
      mask help: Models a lag of the form 1/(b*s+1) where s is the Laplace operator.
  Actuator Dynamics FR : Subsystem  mask(First-order lag supporting vector signals){b=HCU.brkTs, x_initial=0}
      mask prompts: b "Filter time constant"; x_initial "Initial output"
      mask help: Models a lag of the form 1/(b*s+1) where s is the Laplace operator.
  Actuator Dynamics RL : Subsystem  mask(First-order lag supporting vector signals){b=HCU.brkTs, x_initial=0}
      mask prompts: b "Filter time constant"; x_initial "Initial output"
      mask help: Models a lag of the form 1/(b*s+1) where s is the Laplace operator.
  Actuator Dynamics RR : Subsystem  mask(First-order lag supporting vector signals){b=HCU.brkTs, x_initial=0}
      mask prompts: b "Filter time constant"; x_initial "Initial output"
      mask help: Models a lag of the form 1/(b*s+1) where s is the Laplace operator.
  Demux{,1..3} (4 alike) : Demux  Outputs=2
  FL Valve Assembly : Subsystem
  FR Valve Assembly : Subsystem
  RL Valve Assembly : Subsystem
  RR Valve Assembly : Subsystem
  Simulink-PS Converter{,1..7} (8 alike) : nesl_utility/Simulink-PS Converter  PhysicalDomain=network_engine_domain  SubClassName=ps_input  LeftPortType=input  RightPortType=output  PseudoPeriodic=off  Frequencies=[]  NoiseDistribution=none  NoiseParameters=[]  Unit=1  AffineConversion=off  FilteringAndDerivatives=provide  SimscapeFilterOrder=1  InputFilterTimeConstant=0.001  UdotUserProvided=0
  "Brk1 " : PMIOPort  Side=Left
  FR : PMIOPort  Port=2  Side=Right
  FL : PMIOPort  Port=3  Side=Right
  "Brk2 " : PMIOPort  Port=4  Side=Left
  RR : PMIOPort  Port=5  Side=Right
  RL : PMIOPort  Port=6  Side=Right
  wires:
  Demux2/1 -> Simulink-PS Converter/1
  Demux/1 -> Simulink-PS Converter6/1
  In Bus Element2/1 -> Actuator Dynamics FR/1(In)
  Demux2/2 -> Simulink-PS Converter1/1
  Demux3/2 -> Simulink-PS Converter5/1
  Demux1/2 -> Simulink-PS Converter3/1
  Actuator Dynamics FR/1(Out) -> Demux2/1
  Actuator Dynamics FL/1(Out) -> Demux/1
  In Bus Element4/1 -> Actuator Dynamics RR/1(In)
  In Bus Element3/1 -> Actuator Dynamics RL/1(In)
  Demux3/1 -> Simulink-PS Converter4/1
  In Bus Element1/1 -> Actuator Dynamics FL/1(In)
  Demux1/1 -> Simulink-PS Converter2/1
  Actuator Dynamics RR/1(Out) -> Demux1/1
  Demux/2 -> Simulink-PS Converter7/1
  Actuator Dynamics RL/1(Out) -> Demux3/1
  connections:
  "Brk2 "/RConn1 -- RL Valve Assembly/LConn1 -- RR Valve Assembly/LConn3
  FR Valve Assembly/LConn3 -- FL Valve Assembly/LConn1 -- "Brk1 "/RConn1
  RL Valve Assembly/RConn1 -- RL/RConn1
  RR Valve Assembly/LConn2 -- Simulink-PS Converter3/RConn1
  Simulink-PS Converter7/RConn1 -- FL Valve Assembly/LConn3
  RR Valve Assembly/LConn1 -- Simulink-PS Converter2/RConn1
  RR Valve Assembly/RConn1 -- RR/RConn1
  FR Valve Assembly/LConn1 -- Simulink-PS Converter/RConn1
  FR Valve Assembly/RConn1 -- FR/RConn1
  FL Valve Assembly/RConn1 -- FL/RConn1
  FR Valve Assembly/LConn2 -- Simulink-PS Converter1/RConn1
  Simulink-PS Converter4/RConn1 -- RL Valve Assembly/LConn2
  Simulink-PS Converter5/RConn1 -- RL Valve Assembly/LConn3
  Simulink-PS Converter6/RConn1 -- FL Valve Assembly/LConn2

== system sscv_braking_ABS_w_vehicle/Brakes with ABS/FCDB/FLW ==
  CP1 : fl_lib/Isothermal Liquid/Elements/Translational Mechanical Converter (IL)  mech_orientation=1  displacement_spec=foundation.enum.DisplacementSpec.Calculate  x0=0 m  interface_area=fcdb.area m^2  dead_volume=fcdb.deadV m^3  pressure_spec=1  environment_pressure=0.101325 MPa  dynamic_compressibility=simscape.enum.onoff.on  p0=tpc.pRes Pa
      settings: InternalSimscapePortConfiguration="{\"Bottom\":[],\"Left\":[{\"id\":\"A\",\"label\":\"A\",\"type\":\"foundation.isothermal_liquid.isothermal_liquid\"},{\"id\":\"C\",\"label\":\"C\",\"type\":\"foundation.mechanical.translational.translational\"}],\"Right\":[{\"id\":\"R\",\"label\":\"R\",\"type\":\"foundation.mechanical.translational.translational\"}],\"Top\":[]}"
  CP2 : fl_lib/Isothermal Liquid/Elements/Translational Mechanical Converter (IL)  mech_orientation=1  displacement_spec=foundation.enum.DisplacementSpec.Calculate  x0=0 m  interface_area=fcdb.area m^2  dead_volume=fcdb.deadV m^3  pressure_spec=1  environment_pressure=0.101325 MPa  dynamic_compressibility=simscape.enum.onoff.on  p0=tpc.pRes Pa
      settings: InternalSimscapePortConfiguration="{\"Bottom\":[],\"Left\":[{\"id\":\"A\",\"label\":\"A\",\"type\":\"foundation.isothermal_liquid.isothermal_liquid\"},{\"id\":\"C\",\"label\":\"C\",\"type\":\"foundation.mechanical.translational.translational\"}],\"Right\":[{\"id\":\"R\",\"label\":\"R\",\"type\":\"foundation.mechanical.translational.translational\"}],\"Top\":[]}"
  Ideal Force Sensor : fl_lib/Mechanical/Mechanical Sensors/Ideal Force Sensor
  Ideal Force Sensor1 : fl_lib/Mechanical/Mechanical Sensors/Ideal Force Sensor
  Loaded-Contact Rotational Friction : sdl_lib/Brakes & Detents/Rotational/Loaded-Contact Rotational Friction  geometry_model=sdl.enum.friction_geometry.radius  r_eff=fcdb.reffF m  d_o=150 mm  d_i=100 mm  enable_faults=simscape.enum.onoff.off  fault_type=sdl.enum.clutchFault.lock  friction_model=sdl.enum.friction_model_TLU_thermal.fixed  mu_w_vector=[0, 100, 1000] rad/s  temperature_TLU=[280, 300, 320] K  mu_static=fcdb.statFric  mu_static_vector=[.4, .38, .36]  mu_coulomb=fcdb.kinFric  mu_coulomb_vector=[.3, .22, .19]  mu_coulomb_temp_vector=[.3, .28, .25]  mu_coulomb_matrix=[.34, .32, .3; .3, .28, .25; .25, .2, .15]  mu_interp_method=simscape.enum.interpolation.linear  mu_extrap_method=simscape.enum.extrapolation.linear  w_tol=0.01 rad/s  force_min=1 N  mu_visc=fcdb.dampDisk N*m/(rad/s)  initial_state_locked=sdl.enum.initial_lock.unlocked  thermal_mass=50 kJ/K  T_init=300 K
      settings: InternalSimscapePortConfiguration="{\"Bottom\":[],\"Left\":[{\"id\":\"N\",\"label\":\"N\",\"type\":\"input\"},{\"id\":\"B\",\"label\":\"B\",\"type\":\"foundation.mechanical.rotational.rotational\"}],\"Right\":[{\"id\":\"F\",\"label\":\"F\",\"type\":\"foundation.mechanical.rotational.rotational\"}],\"Top\":[]}"
  Mass : fl_lib/Mechanical/Translational Elements/Mass  mass=fcdb.mass kg  num_ports=foundation.enum.numPorts2.one  v_specify=off  v_priority=High  v=0 m/s  v_nominal_specify=off  v_nominal_value=1  v_nominal_unit=m/s  f_specify=off  f_priority=None  f=0 N  f_nominal_specify=off  f_nominal_value=1  f_nominal_unit=N
  Mass1 : fl_lib/Mechanical/Translational Elements/Mass  mass=fcdb.mass kg  num_ports=foundation.enum.numPorts2.one  v_specify=off  v_priority=High  v=0 m/s  v_nominal_specify=off  v_nominal_value=1  v_nominal_unit=m/s  f_specify=off  f_priority=None  f=0 N  f_nominal_specify=off  f_nominal_value=1  f_nominal_unit=N
  Mechanical Rotational Reference : fl_lib/Mechanical/Rotational Elements/Mechanical Rotational Reference
  Mechanical Translational Reference : fl_lib/Mechanical/Translational Elements/Mechanical Translational Reference
  PS Add1 : fl_lib/Physical Signals/Functions/PS Add
  Translational Damper : fl_lib/Mechanical/Translational Elements/Translational Damper  D=fcdb.damp N/(m/s)  v_specify=off  v_priority=None  v=0 m/s  v_nominal_specify=off  v_nominal_value=1  v_nominal_unit=m/s  f_specify=off  f_priority=None  f=0 N  f_nominal_specify=off  f_nominal_value=1  f_nominal_unit=N
  Translational Damper1 : fl_lib/Mechanical/Translational Elements/Translational Damper  D=fcdb.damp N/(m/s)  v_specify=off  v_priority=None  v=0 m/s  v_nominal_specify=off  v_nominal_value=1  v_nominal_unit=m/s  f_specify=off  f_priority=None  f=0 N  f_nominal_specify=off  f_nominal_value=1  f_nominal_unit=N
  Translational Hard Stop : fl_lib/Mechanical/Translational Elements/Translational Hard Stop  upper_bnd=fcdb.runClear m  lower_bnd=0 m  model=simscape.enum.hardstop.smooth  stiff_up=fcdb.complianceF N/m  stiff_low=fcdb.hss N/m  D_up=fcdb.damp N/(m/s)  D_low=fcdb.hsd N/(m/s)  transition=0.1 mm  coeff_rest=0.7  v_tol=0.001 m/s  f_tol=0.001 N  v_specify=off  v_priority=None  v=0 m/s  v_nominal_specify=off  v_nominal_value=1  v_nominal_unit=m/s  f_specify=off  f_priority=None  f=0 N  f_nominal_specify=off  f_nominal_value=1  f_nominal_unit=N  x_specify=off  x_priority=High  x=0 m  x_nominal_specify=off  x_nominal_value=1  x_nominal_unit=m  M_specify=off  M_priority=None  M=0
  Translational Hard Stop1 : fl_lib/Mechanical/Translational Elements/Translational Hard Stop  upper_bnd=fcdb.runClear m  lower_bnd=0 m  model=simscape.enum.hardstop.smooth  stiff_up=fcdb.complianceF N/m  stiff_low=fcdb.hss N/m  D_up=fcdb.damp N/(m/s)  D_low=fcdb.hsd N/(m/s)  transition=0.1 mm  coeff_rest=0.7  v_tol=0.001 m/s  f_tol=0.001 N  v_specify=off  v_priority=None  v=0 m/s  v_nominal_specify=off  v_nominal_value=1  v_nominal_unit=m/s  f_specify=off  f_priority=None  f=0 N  f_nominal_specify=off  f_nominal_value=1  f_nominal_unit=N  x_specify=off  x_priority=High  x=0 m  x_nominal_specify=off  x_nominal_value=1  x_nominal_unit=m  M_specify=off  M_priority=None  M=0
  Brk1 : PMIOPort  Side=Left
  TFLW : PMIOPort  Port=2  Side=Right
  connections:
  Ideal Force Sensor/LConn1 -- Translational Damper/RConn1 -- Translational Hard Stop/RConn1
  Translational Damper1/LConn1 -- CP2/RConn1 -- Mass1/LConn1 -- Translational Hard Stop1/LConn1
  Ideal Force Sensor1/LConn1 -- Translational Damper1/RConn1 -- Translational Hard Stop1/RConn1
  PS Add1/LConn1 -- Ideal Force Sensor/RConn2
  PS Add1/LConn2 -- Ideal Force Sensor1/RConn2
  Loaded-Contact Rotational Friction/LConn1 -- PS Add1/RConn1
  Mechanical Rotational Reference/LConn1 -- Loaded-Contact Rotational Friction/LConn2
  TFLW/RConn1 -- Loaded-Contact Rotational Friction/RConn1
  Translational Damper/LConn1 -- Mass/LConn1 -- CP1/RConn1 -- Translational Hard Stop/LConn1
  Brk1/RConn1 -- CP2/LConn1 -- CP1/LConn1
  Ideal Force Sensor1/RConn1 -- CP2/LConn2 -- Ideal Force Sensor/RConn1 -- CP1/LConn2 -- Mechanical Translational Reference/LConn1

== system sscv_braking_ABS_w_vehicle/Brakes with ABS/FCDB/FRW ==
  CP1 : fl_lib/Isothermal Liquid/Elements/Translational Mechanical Converter (IL)  mech_orientation=1  displacement_spec=foundation.enum.DisplacementSpec.Calculate  x0=0 m  interface_area=fcdb.area m^2  dead_volume=fcdb.deadV m^3  pressure_spec=1  environment_pressure=0.101325 MPa  dynamic_compressibility=simscape.enum.onoff.on  p0=tpc.pRes Pa
      settings: InternalSimscapePortConfiguration="{\"Bottom\":[],\"Left\":[{\"id\":\"A\",\"label\":\"A\",\"type\":\"foundation.isothermal_liquid.isothermal_liquid\"},{\"id\":\"C\",\"label\":\"C\",\"type\":\"foundation.mechanical.translational.translational\"}],\"Right\":[{\"id\":\"R\",\"label\":\"R\",\"type\":\"foundation.mechanical.translational.translational\"}],\"Top\":[]}"
  CP2 : fl_lib/Isothermal Liquid/Elements/Translational Mechanical Converter (IL)  mech_orientation=1  displacement_spec=foundation.enum.DisplacementSpec.Calculate  x0=0 m  interface_area=fcdb.area m^2  dead_volume=fcdb.deadV m^3  pressure_spec=1  environment_pressure=0.101325 MPa  dynamic_compressibility=simscape.enum.onoff.on  p0=tpc.pRes Pa
      settings: InternalSimscapePortConfiguration="{\"Bottom\":[],\"Left\":[{\"id\":\"A\",\"label\":\"A\",\"type\":\"foundation.isothermal_liquid.isothermal_liquid\"},{\"id\":\"C\",\"label\":\"C\",\"type\":\"foundation.mechanical.translational.translational\"}],\"Right\":[{\"id\":\"R\",\"label\":\"R\",\"type\":\"foundation.mechanical.translational.translational\"}],\"Top\":[]}"
  Ideal Force Sensor : fl_lib/Mechanical/Mechanical Sensors/Ideal Force Sensor
  Ideal Force Sensor1 : fl_lib/Mechanical/Mechanical Sensors/Ideal Force Sensor
  Loaded-Contact Rotational Friction : sdl_lib/Brakes & Detents/Rotational/Loaded-Contact Rotational Friction  geometry_model=sdl.enum.friction_geometry.radius  r_eff=fcdb.reffF m  d_o=150 mm  d_i=100 mm  enable_faults=simscape.enum.onoff.off  fault_type=sdl.enum.clutchFault.lock  friction_model=sdl.enum.friction_model_TLU_thermal.fixed  mu_w_vector=[0, 100, 1000] rad/s  temperature_TLU=[280, 300, 320] K  mu_static=fcdb.statFric  mu_static_vector=[.4, .38, .36]  mu_coulomb=fcdb.kinFric  mu_coulomb_vector=[.3, .22, .19]  mu_coulomb_temp_vector=[.3, .28, .25]  mu_coulomb_matrix=[.34, .32, .3; .3, .28, .25; .25, .2, .15]  mu_interp_method=simscape.enum.interpolation.linear  mu_extrap_method=simscape.enum.extrapolation.linear  w_tol=0.01 rad/s  force_min=1 N  mu_visc=fcdb.dampDisk N*m/(rad/s)  initial_state_locked=sdl.enum.initial_lock.unlocked  thermal_mass=50 kJ/K  T_init=300 K
      settings: InternalSimscapePortConfiguration="{\"Bottom\":[],\"Left\":[{\"id\":\"N\",\"label\":\"N\",\"type\":\"input\"},{\"id\":\"B\",\"label\":\"B\",\"type\":\"foundation.mechanical.rotational.rotational\"}],\"Right\":[{\"id\":\"F\",\"label\":\"F\",\"type\":\"foundation.mechanical.rotational.rotational\"}],\"Top\":[]}"
  Mass : fl_lib/Mechanical/Translational Elements/Mass  mass=fcdb.mass kg  num_ports=foundation.enum.numPorts2.one  v_specify=off  v_priority=High  v=0 m/s  v_nominal_specify=off  v_nominal_value=1  v_nominal_unit=m/s  f_specify=off  f_priority=None  f=0 N  f_nominal_specify=off  f_nominal_value=1  f_nominal_unit=N
  Mass1 : fl_lib/Mechanical/Translational Elements/Mass  mass=fcdb.mass kg  num_ports=foundation.enum.numPorts2.one  v_specify=off  v_priority=High  v=0 m/s  v_nominal_specify=off  v_nominal_value=1  v_nominal_unit=m/s  f_specify=off  f_priority=None  f=0 N  f_nominal_specify=off  f_nominal_value=1  f_nominal_unit=N
  Mechanical Rotational Reference : fl_lib/Mechanical/Rotational Elements/Mechanical Rotational Reference
  Mechanical Translational Reference : fl_lib/Mechanical/Translational Elements/Mechanical Translational Reference
  PS Add : fl_lib/Physical Signals/Functions/PS Add
  Translational Damper : fl_lib/Mechanical/Translational Elements/Translational Damper  D=fcdb.damp N/(m/s)  v_specify=off  v_priority=None  v=0 m/s  v_nominal_specify=off  v_nominal_value=1  v_nominal_unit=m/s  f_specify=off  f_priority=None  f=0 N  f_nominal_specify=off  f_nominal_value=1  f_nominal_unit=N
  Translational Damper1 : fl_lib/Mechanical/Translational Elements/Translational Damper  D=fcdb.damp N/(m/s)  v_specify=off  v_priority=None  v=0 m/s  v_nominal_specify=off  v_nominal_value=1  v_nominal_unit=m/s  f_specify=off  f_priority=None  f=0 N  f_nominal_specify=off  f_nominal_value=1  f_nominal_unit=N
  Translational Hard Stop : fl_lib/Mechanical/Translational Elements/Translational Hard Stop  upper_bnd=fcdb.runClear m  lower_bnd=0 m  model=simscape.enum.hardstop.smooth  stiff_up=fcdb.complianceF N/m  stiff_low=fcdb.hss N/m  D_up=fcdb.damp N/(m/s)  D_low=fcdb.hsd N/(m/s)  transition=0.1 mm  coeff_rest=0.7  v_tol=0.001 m/s  f_tol=0.001 N  v_specify=off  v_priority=None  v=0 m/s  v_nominal_specify=off  v_nominal_value=1  v_nominal_unit=m/s  f_specify=off  f_priority=None  f=0 N  f_nominal_specify=off  f_nominal_value=1  f_nominal_unit=N  x_specify=off  x_priority=High  x=0 m  x_nominal_specify=off  x_nominal_value=1  x_nominal_unit=m  M_specify=off  M_priority=None  M=0
  Translational Hard Stop1 : fl_lib/Mechanical/Translational Elements/Translational Hard Stop  upper_bnd=fcdb.runClear m  lower_bnd=0 m  model=simscape.enum.hardstop.smooth  stiff_up=fcdb.complianceF N/m  stiff_low=fcdb.hss N/m  D_up=fcdb.damp N/(m/s)  D_low=fcdb.hsd N/(m/s)  transition=0.1 mm  coeff_rest=0.7  v_tol=0.001 m/s  f_tol=0.001 N  v_specify=off  v_priority=None  v=0 m/s  v_nominal_specify=off  v_nominal_value=1  v_nominal_unit=m/s  f_specify=off  f_priority=None  f=0 N  f_nominal_specify=off  f_nominal_value=1  f_nominal_unit=N  x_specify=off  x_priority=High  x=0 m  x_nominal_specify=off  x_nominal_value=1  x_nominal_unit=m  M_specify=off  M_priority=None  M=0
  Brk1 : PMIOPort  Side=Left
  TFRW : PMIOPort  Port=2  Side=Right
  connections:
  Ideal Force Sensor1/RConn2 -- PS Add/LConn2
  PS Add/LConn1 -- Ideal Force Sensor/RConn2
  Ideal Force Sensor1/LConn1 -- Translational Hard Stop1/RConn1 -- Translational Damper1/RConn1
  Translational Damper/RConn1 -- Translational Hard Stop/RConn1 -- Ideal Force Sensor/LConn1
  PS Add/RConn1 -- Loaded-Contact Rotational Friction/LConn1
  Mechanical Rotational Reference/LConn1 -- Loaded-Contact Rotational Friction/LConn2
  TFRW/RConn1 -- Loaded-Contact Rotational Friction/RConn1
  Translational Damper/LConn1 -- Mass/LConn1 -- CP1/RConn1 -- Translational Hard Stop/LConn1
  Brk1/RConn1 -- CP2/LConn1 -- CP1/LConn1
  Translational Hard Stop1/LConn1 -- Mass1/LConn1 -- CP2/RConn1 -- Translational Damper1/LConn1
  Mechanical Translational Reference/LConn1 -- Ideal Force Sensor1/RConn1 -- CP2/LConn2 -- Ideal Force Sensor/RConn1 -- CP1/LConn2
